simulink model "eight_model_with_R_mod"  (R2022a)
settings: Solver=FixedStepAuto  StartTime=0.0  StopTime=10.0  FixedStep=1e-3  RelTol=1e-3  EnableMultiTasking=on
undefined symbols (not defined in the file): D0, D1, D10, D11, D12, D13, D2, D3, D4, D5, D6, D7, D8, D9, magnitude, PTA0, PTA1, PTA2, PTB23, PTB9, PTC16, PTC17, PTC2, PTC3, PTC4, PTD0, PTD1, PTD2, PTD3
libraries: etargetslib x30, frdmk64flib x18, dspstat3 x1, simulink x1
(part 2 of 2)

== stateflow chart eight_model_with_R_mod/Requirements Table ==
  (default) -> (junction 1073741860)
  (junction 1073741860) -> (junction 1073741861) : {
      | % SF_REQ_REV_07
      | }
  (junction 1073741861) -> (junction 1073741863) : {
      | % HEADER_ASSIGNMENTS
      |
      | }
  (junction 1073741863) -> (junction 1073741865) : {
      | % START_A_4
      | }
  (junction 1073741865) -> (junction 1073741867) : {
      | }
  (junction 1073741867) -> (junction 1073741869)
  (junction 1073741869) -> (junction 1073741871) : {
      | }
  (junction 1073741871) -> (junction 1073741873) : {
      | % END_A_4
      | }
  (junction 1073741873) -> (junction 1073741910) : {
      | % START_R_1
      | }
  (junction 1073741910) -> (junction 1073741912) : {
      | }
  (junction 1073741912) -> (junction 1073741914) : {
      |
      |
      | }
  (junction 1073741914) -> (junction 1073741916) : {
      | }
  (junction 1073741916) -> (junction 1073741944) : {
      | % START_R_7
      | }
  (junction 1073741944) -> (junction 1073741946) : {
      | }
  (junction 1073741946) -> (junction 1073741948)
  (junction 1073741948) -> (junction 1073741950) [order 1] : [(((status) == (0000)))]
  (junction 1073741948) -> (junction 1073741956) [order 2]
  (junction 1073741950) -> (junction 1073741952) : {
      | reqtable_postcondition((((PACE_CHARGE_CTRL) == (1))) && (((Z_ATR_CTRL) == (0))) && (((Z_VENT_CTRL) == (0))) && (((ATR_PACE_CTRL) == (0))) && (((VENT_PACE_CTRL) == (0))) && (((PACE_GND_CTRL) == (1))) && (((ATR_GND_CTRL) == (1))) && (((VENT_GND_CTRL) == (0))) && (((FRONTEND_CTRL) == (0))), 'R:1.1');
      |
      |
      | }
  (junction 1073741952) -> (junction 1073741954) : {
      | }
  (junction 1073741954) -> (junction 1073741956)
  (junction 1073741956) -> (junction 1073741958)
  (junction 1073741958) -> (junction 1073741960) : {
      | % END_R_7
      | }
  (junction 1073741960) -> (junction 1073741965) : {
      | % START_R_10
      | }
  (junction 1073741965) -> (junction 1073741967) : {
      | }
  (junction 1073741967) -> (junction 1073741969)
  (junction 1073741969) -> (junction 1073741971) [order 1] : [(((status) == (0001)))]
  (junction 1073741969) -> (junction 1073741977) [order 2]
  (junction 1073741971) -> (junction 1073741973) : {
      | reqtable_postcondition((((PACE_CHARGE_CTRL) == (0))) && (((Z_ATR_CTRL) == (0))) && (((Z_VENT_CTRL) == (0))) && (((ATR_PACE_CTRL) == (1))) && (((VENT_PACE_CTRL) == (0))) && (((PACE_GND_CTRL) == (1))) && (((ATR_GND_CTRL) == (0))) && (((VENT_GND_CTRL) == (0))) && (((FRONTEND_CTRL) == (0))), 'R:1.2');
      |
      |
      | }
  (junction 1073741973) -> (junction 1073741975) : {
      | }
  (junction 1073741975) -> (junction 1073741977)
  (junction 1073741977) -> (junction 1073741979)
  (junction 1073741979) -> (junction 1073741981) : {
      | % END_R_10
      | }
  (junction 1073741981) -> (junction 1073741928) : {
      | % END_R_1
      | }
  (junction 1073741928) -> (junction 1073741998) : {
      | % START_R_13
      | }
  (junction 1073741998) -> (junction 1073742000) : {
      | }
  (junction 1073742000) -> (junction 1073742002) : {
      |
      |
      | }
  (junction 1073742002) -> (junction 1073742004) : {
      | }
  (junction 1073742004) -> (junction 1073742032) : {
      | % START_R_16
      | }
  (junction 1073742032) -> (junction 1073742034) : {
      | }
  (junction 1073742034) -> (junction 1073742036)
  (junction 1073742036) -> (junction 1073742038) [order 1] : [(((status) == (0010)))]
  (junction 1073742036) -> (junction 1073742044) [order 2]
  (junction 1073742038) -> (junction 1073742040) : {
      | reqtable_postcondition((((PACE_CHARGE_CTRL) == (1))) && (((Z_ATR_CTRL) == (0))) && (((Z_VENT_CTRL) == (0))) && (((ATR_PACE_CTRL) == (0))) && (((VENT_PACE_CTRL) == (0))) && (((PACE_GND_CTRL) == (1))) && (((ATR_GND_CTRL) == (0))) && (((VENT_GND_CTRL) == (1))) && (((FRONTEND_CTRL) == (0))), 'R:2.1');
      |
      |
      | }
  (junction 1073742040) -> (junction 1073742042) : {
      | }
  (junction 1073742042) -> (junction 1073742044)
  (junction 1073742044) -> (junction 1073742046)
  (junction 1073742046) -> (junction 1073742048) : {
      | % END_R_16
      | }
  (junction 1073742048) -> (junction 1073742053) : {
      | % START_R_19
      | }
  (junction 1073742053) -> (junction 1073742055) : {
      | }
  (junction 1073742055) -> (junction 1073742057)
  (junction 1073742057) -> (junction 1073742059) [order 1] : [(((status) == (0011)))]
  (junction 1073742057) -> (junction 1073742065) [order 2]
  (junction 1073742059) -> (junction 1073742061) : {
      | reqtable_postcondition((((PACE_CHARGE_CTRL) == (0))) && (((Z_ATR_CTRL) == (0))) && (((Z_VENT_CTRL) == (0))) && (((ATR_PACE_CTRL) == (0))) && (((VENT_PACE_CTRL) == (0))) && (((PACE_GND_CTRL) == (1))) && (((ATR_GND_CTRL) == (0))) && (((VENT_GND_CTRL) == (0))) && (((FRONTEND_CTRL) == (0))), 'R:2.2');
      |
      |
      | }
  (junction 1073742061) -> (junction 1073742063) : {
      | }
  (junction 1073742063) -> (junction 1073742065)
  (junction 1073742065) -> (junction 1073742067)
  (junction 1073742067) -> (junction 1073742069) : {
      | % END_R_19
      | }
  (junction 1073742069) -> (junction 1073742016) : {
      | % END_R_13
      | }
  (junction 1073742016) -> (junction 1073742086) : {
      | % START_R_22
      | }
  (junction 1073742086) -> (junction 1073742088) : {
      | }
  (junction 1073742088) -> (junction 1073742090) : {
      |
      |
      | }
  (junction 1073742090) -> (junction 1073742092) : {
      | }
  (junction 1073742092) -> (junction 1073742200) : {
      | % START_R_25
      | }
  (junction 1073742200) -> (junction 1073742202) : {
      | }
  (junction 1073742202) -> (junction 1073742204)
  (junction 1073742204) -> (junction 1073742206) [order 1] : [(((status) == (0100)))]
  (junction 1073742204) -> (junction 1073742212) [order 2]
  (junction 1073742206) -> (junction 1073742208) : {
      | reqtable_postcondition((((PACE_CHARGE_CTRL) == (1))) && (((Z_ATR_CTRL) == (0))) && (((Z_VENT_CTRL) == (0))) && (((ATR_PACE_CTRL) == (0))) && (((VENT_PACE_CTRL) == (0))) && (((PACE_GND_CTRL) == (1))) && (((ATR_GND_CTRL) == (1))) && (((VENT_GND_CTRL) == (0))) && (((FRONTEND_CTRL) == (1))), 'R:3.1');
      |
      |
      | }
  (junction 1073742208) -> (junction 1073742210) : {
      | }
  (junction 1073742210) -> (junction 1073742212)
  (junction 1073742212) -> (junction 1073742214)
  (junction 1073742214) -> (junction 1073742216) : {
      | % END_R_25
      | }
  (junction 1073742216) -> (junction 1073742221) : {
      | % START_R_28
      | }
  (junction 1073742221) -> (junction 1073742223) : {
      | }
  (junction 1073742223) -> (junction 1073742225)
  (junction 1073742225) -> (junction 1073742227) [order 1] : [(((status) == (0101)))]
  (junction 1073742225) -> (junction 1073742233) [order 2]
  (junction 1073742227) -> (junction 1073742229) : {
      | reqtable_postcondition((((PACE_CHARGE_CTRL) == (1))) && (((Z_ATR_CTRL) == (0))) && (((Z_VENT_CTRL) == (0))) && (((ATR_PACE_CTRL) == (0))) && (((VENT_PACE_CTRL) == (0))) && (((PACE_GND_CTRL) == (1))) && (((ATR_GND_CTRL) == (1))) && (((VENT_GND_CTRL) == (0))) && (((FRONTEND_CTRL) == (1))), 'R:3.2');
      |
      |
      | }
  (junction 1073742229) -> (junction 1073742231) : {
      | }
  (junction 1073742231) -> (junction 1073742233)
  (junction 1073742233) -> (junction 1073742235)
  (junction 1073742235) -> (junction 1073742237) : {
      | % END_R_28
      | }
  (junction 1073742237) -> (junction 1073742242) : {
      | % START_R_31
      | }
  (junction 1073742242) -> (junction 1073742244) : {
      | }
  (junction 1073742244) -> (junction 1073742246)
  (junction 1073742246) -> (junction 1073742248) [order 1] : [(((status) == (0110)))]
  (junction 1073742246) -> (junction 1073742254) [order 2]
  (junction 1073742248) -> (junction 1073742250) : {
      | reqtable_postcondition((((PACE_CHARGE_CTRL) == (0))) && (((Z_ATR_CTRL) == (0))) && (((Z_VENT_CTRL) == (0))) && (((ATR_PACE_CTRL) == (1))) && (((VENT_PACE_CTRL) == (0))) && (((PACE_GND_CTRL) == (1))) && (((ATR_GND_CTRL) == (0))) && (((VENT_GND_CTRL) == (0))) && (((FRONTEND_CTRL) == (1))), 'R:3.3');
      |
      |
      | }
  (junction 1073742250) -> (junction 1073742252) : {
      | }
  (junction 1073742252) -> (junction 1073742254)
  (junction 1073742254) -> (junction 1073742256)
  (junction 1073742256) -> (junction 1073742258) : {
      | % END_R_31
      | }
  (junction 1073742258) -> (junction 1073742104) : {
      | % END_R_22
      | }
  (junction 1073742104) -> (junction 1073742275) : {
      | % START_R_34
      | }
  (junction 1073742275) -> (junction 1073742277) : {
      | }
  (junction 1073742277) -> (junction 1073742279) : {
      |
      |
      | }
  (junction 1073742279) -> (junction 1073742281) : {
      | }
  (junction 1073742281) -> (junction 1073742321) : {
      | % START_R_37
      | }
  (junction 1073742321) -> (junction 1073742323) : {
      | }
  (junction 1073742323) -> (junction 1073742325)
  (junction 1073742325) -> (junction 1073742327) [order 1] : [(((status) == (0111)))]
  (junction 1073742325) -> (junction 1073742333) [order 2]
  (junction 1073742327) -> (junction 1073742329) : {
      | reqtable_postcondition((((PACE_CHARGE_CTRL) == (1))) && (((Z_ATR_CTRL) == (0))) && (((Z_VENT_CTRL) == (0))) && (((ATR_PACE_CTRL) == (0))) && (((VENT_PACE_CTRL) == (0))) && (((PACE_GND_CTRL) == (1))) && (((ATR_GND_CTRL) == (0))) && (((VENT_GND_CTRL) == (1))) && (((FRONTEND_CTRL) == (1))), 'R:4.1');
      |
      |
      | }
  (junction 1073742329) -> (junction 1073742331) : {
      | }
  (junction 1073742331) -> (junction 1073742333)
  (junction 1073742333) -> (junction 1073742335)
  (junction 1073742335) -> (junction 1073742337) : {
      | % END_R_37
      | }
  (junction 1073742337) -> (junction 1073742342) : {
      | % START_R_40
      | }
  (junction 1073742342) -> (junction 1073742344) : {
      | }
  (junction 1073742344) -> (junction 1073742346)
  (junction 1073742346) -> (junction 1073742348) [order 1] : [(((status) == (1000)))]
  (junction 1073742346) -> (junction 1073742354) [order 2]
  (junction 1073742348) -> (junction 1073742350) : {
      | reqtable_postcondition((((PACE_CHARGE_CTRL) == (1))) && (((Z_ATR_CTRL) == (0))) && (((Z_VENT_CTRL) == (0))) && (((ATR_PACE_CTRL) == (0))) && (((VENT_PACE_CTRL) == (0))) && (((PACE_GND_CTRL) == (1))) && (((ATR_GND_CTRL) == (0))) && (((VENT_GND_CTRL) == (1))) && (((FRONTEND_CTRL) == (1))), 'R:4.2');
      |
      |
      | }
  (junction 1073742350) -> (junction 1073742352) : {
      | }
  (junction 1073742352) -> (junction 1073742354)
  (junction 1073742354) -> (junction 1073742356)
  (junction 1073742356) -> (junction 1073742358) : {
      | % END_R_40
      | }
  (junction 1073742358) -> (junction 1073742363) : {
      | % START_R_43
      | }
  (junction 1073742363) -> (junction 1073742365) : {
      | }
  (junction 1073742365) -> (junction 1073742367)
  (junction 1073742367) -> (junction 1073742369) [order 1] : [(((status) == (1001)))]
  (junction 1073742367) -> (junction 1073742375) [order 2]
  (junction 1073742369) -> (junction 1073742371) : {
      | reqtable_postcondition((((PACE_CHARGE_CTRL) == (0))) && (((Z_ATR_CTRL) == (0))) && (((Z_VENT_CTRL) == (0))) && (((ATR_PACE_CTRL) == (0))) && (((VENT_PACE_CTRL) == (1))) && (((PACE_GND_CTRL) == (1))) && (((ATR_GND_CTRL) == (0))) && (((VENT_GND_CTRL) == (0))) && (((FRONTEND_CTRL) == (1))), 'R:4.3');
      |
      |
      | }
  (junction 1073742371) -> (junction 1073742373) : {
      | }
  (junction 1073742373) -> (junction 1073742375)
  (junction 1073742375) -> (junction 1073742377)
  (junction 1073742377) -> (junction 1073742379) : {
      | % END_R_43
      | }
  (junction 1073742379) -> (junction 1073742293) : {
      | % END_R_34
      | }
  data: ATR_GND_CTRL input; ATR_PACE_CTRL input; VENT_GND_CTRL input; VENT_PACE_CTRL input; Z_ATR_CTRL input; Z_VENT_CTRL input; FRONTEND_CTRL input; PACE_GND_CTRL input; PACE_CHARGE_CTRL input; status input
